simulink library "batt_packBTMSExampleLib"  (R2023a)
settings: Solver=VariableStepAuto  StartTime=0.0  StopTime=10.0  RelTol=1e-3
libraries: batt_packBTMSExampleLib_lib x12
(part 1 of 2)
settings Model: Creator=jjha  LastModifiedBy=jjha
settings OptimizationCC: ReuseModelBlockBuffer=off

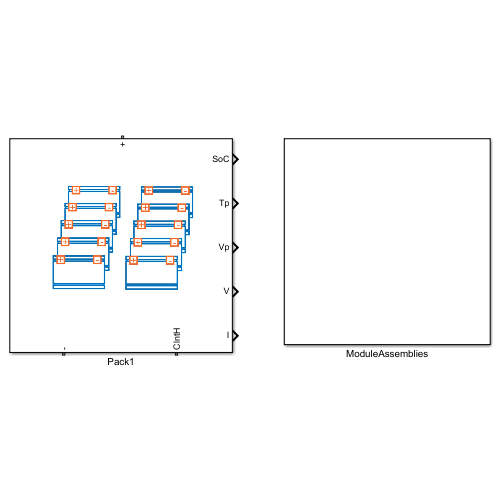
[thumbnail: Simulink's stored preview of the top-level diagram]
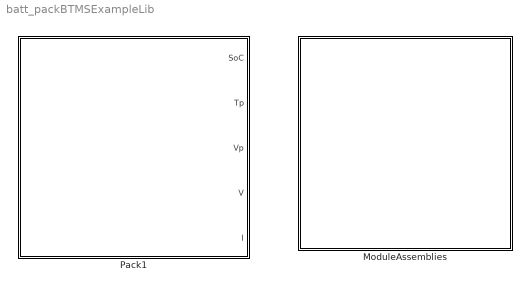
== system batt_packBTMSExampleLib ==
  ModuleAssemblies : Subsystem
  Pack1 : Subsystem
      settings: CopyFcn=set_param(gcb, 'LinkStatus', 'breakWithoutHierarchy')  PortSchema="{\"entries\":[{\"content\":{\"sides\":[{\"content\":{\"connectorIds\":[\"LConn1\"]},\"type\":\"ConnectorPlacement.EquallySpacedRectSide\",\"uuid\":\"7b46babc-8b83-451b-8519-1d7c62ae3771\"},{\"content\":{\"connectorIds\":[\"RConn1\",\"RConn2\"],\"side\":\"RIGHT\"},\"type\":\"ConnectorPlacement.EquallySpacedRectSide\",\"uuid\":\"75c1bf7b-5e52-4279-86bf-85530d236c02\"},{\"content\":{\"connectorIds\":[],\"side\":\"TOP\"},\"type\":\"ConnectorPlacement.EquallySpacedRectSide\",\"uuid\":\"90212396-c9c9-431a-bb2e-a5c41a4990d7\"},{\"content\":{\"connectorIds\":[\"Out1\",\"Out2\",\"Out3\",\"Out4\",\"Out5\"],\"side\":\"BOTTOM\"},\"type\":\"ConnectorPlacement.EquallySpacedRectSide\",\"uuid\":\"256631cd-ebba-4ea5-bbad-0309b84a78ed\"}]},\"type\":\"ConnectorPlacement.EquallySpacedConnector\",\"uuid\":\"fb66d0bc-bd1f-4bb9-a18e-b6b74cdcb9a0\"}],\"packageUris\":[\"http://schema.mathworks.com/mf0/Connector/R2020b\"],\"version\":\"1.0\"}"
      mask Display: image('$imagefile')

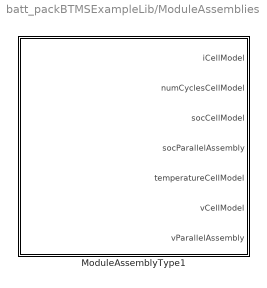
== system batt_packBTMSExampleLib/ModuleAssemblies ==
  ModuleAssemblyType1 : Subsystem
      settings: CopyFcn=set_param(gcb, 'LinkStatus', 'breakWithoutHierarchy')  PortSchema="{\"entries\":[{\"content\":{\"sides\":[{\"content\":{\"connectorIds\":[\"LConn1\"]},\"type\":\"ConnectorPlacement.EquallySpacedRectSide\",\"uuid\":\"7b46babc-8b83-451b-8519-1d7c62ae3771\"},{\"content\":{\"connectorIds\":[\"RConn1\",\"RConn2\"],\"side\":\"RIGHT\"},\"type\":\"ConnectorPlacement.EquallySpacedRectSide\",\"uuid\":\"75c1bf7b-5e52-4279-86bf-85530d236c02\"},{\"content\":{\"connectorIds\":[],\"side\":\"TOP\"},\"type\":\"ConnectorPlacement.EquallySpacedRectSide\",\"uuid\":\"90212396-c9c9-431a-bb2e-a5c41a4990d7\"},{\"content\":{\"connectorIds\":[\"Out1\",\"Out2\",\"Out3\",\"Out4\",\"Out5\",\"Out6\",\"Out7\"],\"side\":\"BOTTOM\"},\"type\":\"ConnectorPlacement.EquallySpacedRectSide\",\"uuid\":\"06be32c4-8297-416c-9a62-5fc7a23f864d\"}]},\"type\":\"ConnectorPlacement.EquallySpacedConnector\",\"uuid\":\"fb66d0bc-bd1f-4bb9-a18e-b6b74cdcb9a0\"}],\"packageUris\":[\"http://schema.mathworks.com/mf0/Connector/R2020b\"],\"version\":\"1.0\"}"
      mask Display: image('$imagefile')

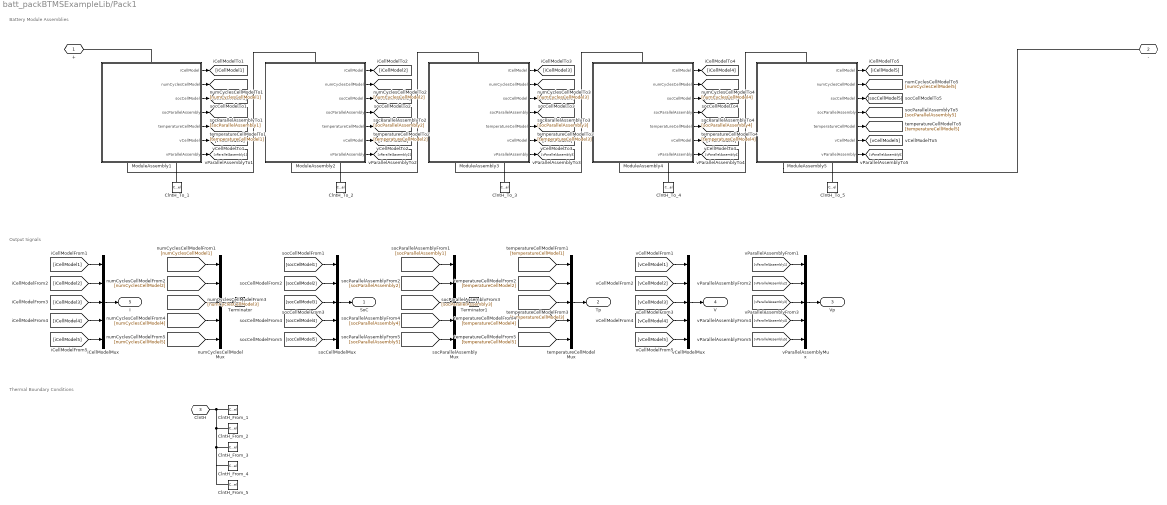
== system batt_packBTMSExampleLib/Pack1 ==
  note: Battery Module Assemblies
  note: Output Signals
  note: Thermal Boundary Conditions
  ClntH_From_1 : ConnectionLabel  Label=clntH_1
  ClntH_From_2 : ConnectionLabel  Label=clntH_2
  ClntH_From_3 : ConnectionLabel  Label=clntH_3
  ClntH_From_4 : ConnectionLabel  Label=clntH_4
  ClntH_From_5 : ConnectionLabel  Label=clntH_5
  ClntH_To_1 : ConnectionLabel  Label=clntH_1
  ClntH_To_2 : ConnectionLabel  Label=clntH_2
  ClntH_To_3 : ConnectionLabel  Label=clntH_3
  ClntH_To_4 : ConnectionLabel  Label=clntH_4
  ClntH_To_5 : ConnectionLabel  Label=clntH_5
  ModuleAssembly1 : Subsystem
      settings: CopyFcn=set_param(gcb, 'LinkStatus', 'breakWithoutHierarchy')  PortSchema="{\"entries\":[{\"content\":{\"sides\":[{\"content\":{\"connectorIds\":[\"LConn1\"]},\"type\":\"ConnectorPlacement.EquallySpacedRectSide\",\"uuid\":\"7b46babc-8b83-451b-8519-1d7c62ae3771\"},{\"content\":{\"connectorIds\":[\"RConn1\",\"RConn2\"],\"side\":\"RIGHT\"},\"type\":\"ConnectorPlacement.EquallySpacedRectSide\",\"uuid\":\"75c1bf7b-5e52-4279-86bf-85530d236c02\"},{\"content\":{\"connectorIds\":[],\"side\":\"TOP\"},\"type\":\"ConnectorPlacement.EquallySpacedRectSide\",\"uuid\":\"90212396-c9c9-431a-bb2e-a5c41a4990d7\"},{\"content\":{\"connectorIds\":[\"Out1\",\"Out2\",\"Out3\",\"Out4\",\"Out5\",\"Out6\",\"Out7\"],\"side\":\"BOTTOM\"},\"type\":\"ConnectorPlacement.EquallySpacedRectSide\",\"uuid\":\"06be32c4-8297-416c-9a62-5fc7a23f864d\"}]},\"type\":\"ConnectorPlacement.EquallySpacedConnector\",\"uuid\":\"fb66d0bc-bd1f-4bb9-a18e-b6b74cdcb9a0\"}],\"packageUris\":[\"http://schema.mathworks.com/mf0/Connector/R2020b\"],\"version\":\"1.0\"}"
      mask Display: image('$imagefile')
  ModuleAssembly2 : Subsystem
      settings: CopyFcn=set_param(gcb, 'LinkStatus', 'breakWithoutHierarchy')  PortSchema="{\"entries\":[{\"content\":{\"sides\":[{\"content\":{\"connectorIds\":[\"LConn1\"]},\"type\":\"ConnectorPlacement.EquallySpacedRectSide\",\"uuid\":\"7b46babc-8b83-451b-8519-1d7c62ae3771\"},{\"content\":{\"connectorIds\":[\"RConn1\",\"RConn2\"],\"side\":\"RIGHT\"},\"type\":\"ConnectorPlacement.EquallySpacedRectSide\",\"uuid\":\"75c1bf7b-5e52-4279-86bf-85530d236c02\"},{\"content\":{\"connectorIds\":[],\"side\":\"TOP\"},\"type\":\"ConnectorPlacement.EquallySpacedRectSide\",\"uuid\":\"90212396-c9c9-431a-bb2e-a5c41a4990d7\"},{\"content\":{\"connectorIds\":[\"Out1\",\"Out2\",\"Out3\",\"Out4\",\"Out5\",\"Out6\",\"Out7\"],\"side\":\"BOTTOM\"},\"type\":\"ConnectorPlacement.EquallySpacedRectSide\",\"uuid\":\"06be32c4-8297-416c-9a62-5fc7a23f864d\"}]},\"type\":\"ConnectorPlacement.EquallySpacedConnector\",\"uuid\":\"fb66d0bc-bd1f-4bb9-a18e-b6b74cdcb9a0\"}],\"packageUris\":[\"http://schema.mathworks.com/mf0/Connector/R2020b\"],\"version\":\"1.0\"}"
      mask Display: image('$imagefile')
  ModuleAssembly3 : Subsystem
      settings: CopyFcn=set_param(gcb, 'LinkStatus', 'breakWithoutHierarchy')  PortSchema="{\"entries\":[{\"content\":{\"sides\":[{\"content\":{\"connectorIds\":[\"LConn1\"]},\"type\":\"ConnectorPlacement.EquallySpacedRectSide\",\"uuid\":\"7b46babc-8b83-451b-8519-1d7c62ae3771\"},{\"content\":{\"connectorIds\":[\"RConn1\",\"RConn2\"],\"side\":\"RIGHT\"},\"type\":\"ConnectorPlacement.EquallySpacedRectSide\",\"uuid\":\"75c1bf7b-5e52-4279-86bf-85530d236c02\"},{\"content\":{\"connectorIds\":[],\"side\":\"TOP\"},\"type\":\"ConnectorPlacement.EquallySpacedRectSide\",\"uuid\":\"90212396-c9c9-431a-bb2e-a5c41a4990d7\"},{\"content\":{\"connectorIds\":[\"Out1\",\"Out2\",\"Out3\",\"Out4\",\"Out5\",\"Out6\",\"Out7\"],\"side\":\"BOTTOM\"},\"type\":\"ConnectorPlacement.EquallySpacedRectSide\",\"uuid\":\"06be32c4-8297-416c-9a62-5fc7a23f864d\"}]},\"type\":\"ConnectorPlacement.EquallySpacedConnector\",\"uuid\":\"fb66d0bc-bd1f-4bb9-a18e-b6b74cdcb9a0\"}],\"packageUris\":[\"http://schema.mathworks.com/mf0/Connector/R2020b\"],\"version\":\"1.0\"}"
      mask Display: image('$imagefile')
  ModuleAssembly4 : Subsystem
      settings: CopyFcn=set_param(gcb, 'LinkStatus', 'breakWithoutHierarchy')  PortSchema="{\"entries\":[{\"content\":{\"sides\":[{\"content\":{\"connectorIds\":[\"LConn1\"]},\"type\":\"ConnectorPlacement.EquallySpacedRectSide\",\"uuid\":\"7b46babc-8b83-451b-8519-1d7c62ae3771\"},{\"content\":{\"connectorIds\":[\"RConn1\",\"RConn2\"],\"side\":\"RIGHT\"},\"type\":\"ConnectorPlacement.EquallySpacedRectSide\",\"uuid\":\"75c1bf7b-5e52-4279-86bf-85530d236c02\"},{\"content\":{\"connectorIds\":[],\"side\":\"TOP\"},\"type\":\"ConnectorPlacement.EquallySpacedRectSide\",\"uuid\":\"90212396-c9c9-431a-bb2e-a5c41a4990d7\"},{\"content\":{\"connectorIds\":[\"Out1\",\"Out2\",\"Out3\",\"Out4\",\"Out5\",\"Out6\",\"Out7\"],\"side\":\"BOTTOM\"},\"type\":\"ConnectorPlacement.EquallySpacedRectSide\",\"uuid\":\"06be32c4-8297-416c-9a62-5fc7a23f864d\"}]},\"type\":\"ConnectorPlacement.EquallySpacedConnector\",\"uuid\":\"fb66d0bc-bd1f-4bb9-a18e-b6b74cdcb9a0\"}],\"packageUris\":[\"http://schema.mathworks.com/mf0/Connector/R2020b\"],\"version\":\"1.0\"}"
      mask Display: image('$imagefile')
  ModuleAssembly5 : Subsystem
      settings: CopyFcn=set_param(gcb, 'LinkStatus', 'breakWithoutHierarchy')  PortSchema="{\"entries\":[{\"content\":{\"sides\":[{\"content\":{\"connectorIds\":[\"LConn1\"]},\"type\":\"ConnectorPlacement.EquallySpacedRectSide\",\"uuid\":\"7b46babc-8b83-451b-8519-1d7c62ae3771\"},{\"content\":{\"connectorIds\":[\"RConn1\",\"RConn2\"],\"side\":\"RIGHT\"},\"type\":\"ConnectorPlacement.EquallySpacedRectSide\",\"uuid\":\"75c1bf7b-5e52-4279-86bf-85530d236c02\"},{\"content\":{\"connectorIds\":[],\"side\":\"TOP\"},\"type\":\"ConnectorPlacement.EquallySpacedRectSide\",\"uuid\":\"90212396-c9c9-431a-bb2e-a5c41a4990d7\"},{\"content\":{\"connectorIds\":[\"Out1\",\"Out2\",\"Out3\",\"Out4\",\"Out5\",\"Out6\",\"Out7\"],\"side\":\"BOTTOM\"},\"type\":\"ConnectorPlacement.EquallySpacedRectSide\",\"uuid\":\"06be32c4-8297-416c-9a62-5fc7a23f864d\"}]},\"type\":\"ConnectorPlacement.EquallySpacedConnector\",\"uuid\":\"fb66d0bc-bd1f-4bb9-a18e-b6b74cdcb9a0\"}],\"packageUris\":[\"http://schema.mathworks.com/mf0/Connector/R2020b\"],\"version\":\"1.0\"}"
      mask Display: image('$imagefile')
  Terminator : Terminator
  Terminator1 : Terminator
  iCellModelMux : Mux  Inputs=5
  numCyclesCellModelMux : Mux  Inputs=5
  socCellModelMux : Mux  Inputs=5
  socParallelAssemblyMux : Mux  Inputs=5
  temperatureCellModelMux : Mux  Inputs=5
  vCellModelMux : Mux  Inputs=5
  vParallelAssemblyMux : Mux  Inputs=5
  + : PMIOPort  Side=Left
  - : PMIOPort  Port=2  Side=Right
  ClntH : PMIOPort  Port=3  Side=Right  ConnectionType=Connection: foundation.thermal.thermal
  SoC : Outport
  Tp : Outport  Port=2
  Vp : Outport  Port=3
  V : Outport  Port=4
  I : Outport  Port=5
  wires:
  ModuleAssembly1/1(iCellModel) -> [iCellModel1]
  iCellModelMux/1 -> I/1
  [iCellModel1] -> iCellModelMux/1
  ModuleAssembly1/2(numCyclesCellModel) -> [numCyclesCellModel1]
  numCyclesCellModelMux/1 -> Terminator/1
  [numCyclesCellModel1] -> numCyclesCellModelMux/1
  ModuleAssembly1/3(socCellModel) -> [socCellModel1]
  socCellModelMux/1 -> SoC/1
  [socCellModel1] -> socCellModelMux/1
  ModuleAssembly1/4(socParallelAssembly) -> [socParallelAssembly1]
  socParallelAssemblyMux/1 -> Terminator1/1
  [socParallelAssembly1] -> socParallelAssemblyMux/1
  ModuleAssembly1/5(temperatureCellModel) -> [temperatureCellModel1]
  temperatureCellModelMux/1 -> Tp/1
  [temperatureCellModel1] -> temperatureCellModelMux/1
  ModuleAssembly1/6(vCellModel) -> [vCellModel1]
  vCellModelMux/1 -> V/1
  [vCellModel1] -> vCellModelMux/1
  ModuleAssembly1/7(vParallelAssembly) -> [vParallelAssembly1]
  vParallelAssemblyMux/1 -> Vp/1
  [vParallelAssembly1] -> vParallelAssemblyMux/1
  ModuleAssembly2/1(iCellModel) -> [iCellModel2]
  [iCellModel2] -> iCellModelMux/2
  ModuleAssembly2/2(numCyclesCellModel) -> [numCyclesCellModel2]
  [numCyclesCellModel2] -> numCyclesCellModelMux/2
  ModuleAssembly2/3(socCellModel) -> [socCellModel2]
  [socCellModel2] -> socCellModelMux/2
  ModuleAssembly2/4(socParallelAssembly) -> [socParallelAssembly2]
  [socParallelAssembly2] -> socParallelAssemblyMux/2
  ModuleAssembly2/5(temperatureCellModel) -> [temperatureCellModel2]
  [temperatureCellModel2] -> temperatureCellModelMux/2
  ModuleAssembly2/6(vCellModel) -> [vCellModel2]
  [vCellModel2] -> vCellModelMux/2
  ModuleAssembly2/7(vParallelAssembly) -> [vParallelAssembly2]
  [vParallelAssembly2] -> vParallelAssemblyMux/2
  ModuleAssembly3/1(iCellModel) -> [iCellModel3]
  [iCellModel3] -> iCellModelMux/3
  ModuleAssembly3/2(numCyclesCellModel) -> [numCyclesCellModel3]
  [numCyclesCellModel3] -> numCyclesCellModelMux/3
  ModuleAssembly3/3(socCellModel) -> [socCellModel3]
  [socCellModel3] -> socCellModelMux/3
  ModuleAssembly3/4(socParallelAssembly) -> [socParallelAssembly3]
  [socParallelAssembly3] -> socParallelAssemblyMux/3
  ModuleAssembly3/5(temperatureCellModel) -> [temperatureCellModel3]
  [temperatureCellModel3] -> temperatureCellModelMux/3
  ModuleAssembly3/6(vCellModel) -> [vCellModel3]
  [vCellModel3] -> vCellModelMux/3
  ModuleAssembly3/7(vParallelAssembly) -> [vParallelAssembly3]
  [vParallelAssembly3] -> vParallelAssemblyMux/3
  ModuleAssembly4/1(iCellModel) -> [iCellModel4]
  [iCellModel4] -> iCellModelMux/4
  ModuleAssembly4/2(numCyclesCellModel) -> [numCyclesCellModel4]
  [numCyclesCellModel4] -> numCyclesCellModelMux/4
  ModuleAssembly4/3(socCellModel) -> [socCellModel4]
  [socCellModel4] -> socCellModelMux/4
  ModuleAssembly4/4(socParallelAssembly) -> [socParallelAssembly4]
  [socParallelAssembly4] -> socParallelAssemblyMux/4
  ModuleAssembly4/5(temperatureCellModel) -> [temperatureCellModel4]
  [temperatureCellModel4] -> temperatureCellModelMux/4
  ModuleAssembly4/6(vCellModel) -> [vCellModel4]
  [vCellModel4] -> vCellModelMux/4
  ModuleAssembly4/7(vParallelAssembly) -> [vParallelAssembly4]
  [vParallelAssembly4] -> vParallelAssemblyMux/4
  ModuleAssembly5/1(iCellModel) -> [iCellModel5]
  [iCellModel5] -> iCellModelMux/5
  ModuleAssembly5/2(numCyclesCellModel) -> [numCyclesCellModel5]
  [numCyclesCellModel5] -> numCyclesCellModelMux/5
  ModuleAssembly5/3(socCellModel) -> [socCellModel5]
  [socCellModel5] -> socCellModelMux/5
  ModuleAssembly5/4(socParallelAssembly) -> [socParallelAssembly5]
  [socParallelAssembly5] -> socParallelAssemblyMux/5
  ModuleAssembly5/5(temperatureCellModel) -> [temperatureCellModel5]
  [temperatureCellModel5] -> temperatureCellModelMux/5
  ModuleAssembly5/6(vCellModel) -> [vCellModel5]
  [vCellModel5] -> vCellModelMux/5
  ModuleAssembly5/7(vParallelAssembly) -> [vParallelAssembly5]
  [vParallelAssembly5] -> vParallelAssemblyMux/5
  connections:
  ModuleAssembly2/LConn1 -- ModuleAssembly1/RConn1
  ModuleAssembly3/LConn1 -- ModuleAssembly2/RConn1
  ModuleAssembly4/LConn1 -- ModuleAssembly3/RConn1
  ModuleAssembly5/LConn1 -- ModuleAssembly4/RConn1
  ModuleAssembly1/LConn1 -- +/RConn1
  ModuleAssembly5/RConn1 -- -/RConn1
  ClntH_To_1/LConn1 -- ModuleAssembly1/RConn2
  ClntH_From_1/LConn1 -- ClntH_From_5/LConn1 -- ClntH_From_4/LConn1 -- ClntH_From_3/LConn1 -- ClntH_From_2/LConn1 -- ClntH/RConn1
  ClntH_To_2/LConn1 -- ModuleAssembly2/RConn2
  ClntH_To_3/LConn1 -- ModuleAssembly3/RConn2
  ClntH_To_4/LConn1 -- ModuleAssembly4/RConn2
  ClntH_To_5/LConn1 -- ModuleAssembly5/RConn2

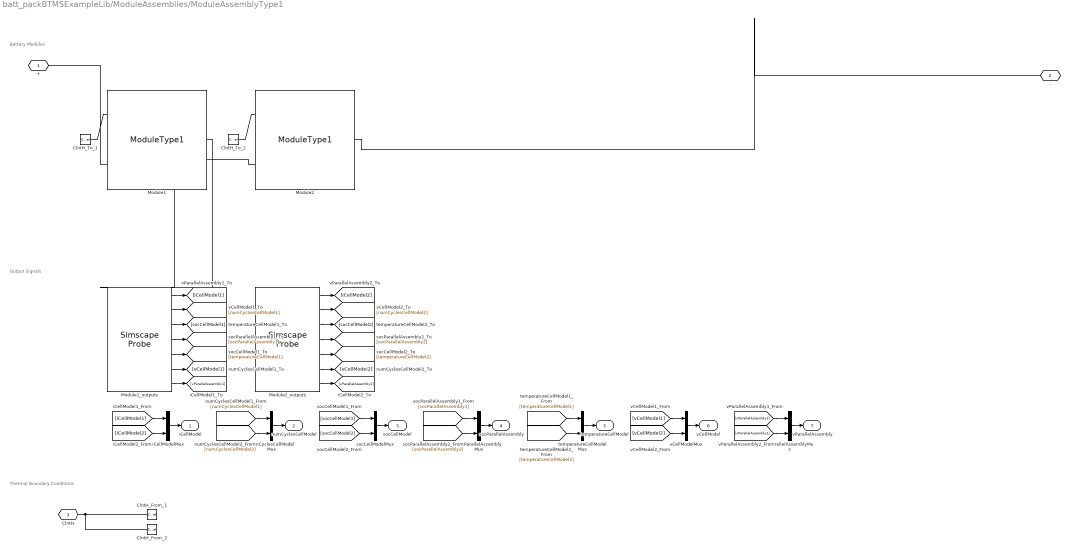
== system batt_packBTMSExampleLib/ModuleAssemblies/ModuleAssemblyType1 ==
  note: Battery Modules
  note: Output Signals
  note: Thermal Boundary Conditions
  ClntH_From_1 : ConnectionLabel  Label=clntH_1
  ClntH_From_2 : ConnectionLabel  Label=clntH_2
  ClntH_To_1 : ConnectionLabel  Label=clntH_1
  ClntH_To_2 : ConnectionLabel  Label=clntH_2
  Module1 : batt_packBTMSExampleLib_lib/Modules/ModuleType1  SOC_vec=ModuleType1.SOC_vec  T_vec=ModuleType1.T_vec K  V0_mat=ModuleType1.V0_mat V  V_range=ModuleType1.V_range V  R0_mat=ModuleType1.R0_mat Ohm  AH=ModuleType1.AH A*hr  extrapolation_option=simscape.enum.extrapolation.nearest  thermal_mass=ModuleType1.thermal_mass J/K  CoolantThermalPathResistance=ModuleType1.CoolantThermalPathResistance K/W  P=3  S=11  iCellModel_specify=off  iCellModel_priority=None  iCellModel=0 A  iCellModel_nominal_specify=off  iCellModel_nominal_unit=A  iCellModel_nominal_value=1  vCellModel_specify=off  vCellModel_priority=None  vCellModel=0 V  vCellModel_nominal_specify=off  vCellModel_nominal_unit=V  vCellModel_nominal_value=1  socCellModel_specify=off  socCellModel_priority=High  socCellModel=1  socCellModel_nominal_specify=off  socCellModel_nominal_unit=1  socCellModel_nominal_value=1  numCyclesCellModel_specify=off  numCyclesCellModel_priority=High  numCyclesCellModel=0  numCyclesCellModel_nominal_specify=off  numCyclesCellModel_nominal_unit=1  numCyclesCellModel_nominal_value=1  temperatureCellModel_specify=off  temperatureCellModel_priority=High  temperatureCellModel=298.15 K  temperatureCellModel_nominal_specify=off  temperatureCellModel_nominal_unit=K  temperatureCellModel_nominal_value=1  vParallelAssembly_specify=off  vParallelAssembly_priority=None  vParallelAssembly=repmat(0, 11, 1) V  vParallelAssembly_nominal_specify=off  vParallelAssembly_nominal_unit=V  vParallelAssembly_nominal_value=1  socParallelAssembly_specify=off  socParallelAssembly_priority=None  socParallelAssembly=repmat(1, 11, 1)  socParallelAssembly_nominal_specify=off  socParallelAssembly_nominal_unit=1  socParallelAssembly_nominal_value=1
      settings: InternalSimscapePortConfiguration="{\"Bottom\":[{\"id\":\"n\",\"label\":\"-\",\"type\":\"foundation.electrical.electrical\"}],\"Left\":[{\"id\":\"ClntH\",\"label\":\"CH\",\"type\":\"foundation.thermal.thermal\"}],\"Right\":[],\"Top\":[{\"id\":\"p\",\"label\":\"+\",\"type\":\"foundation.electrical.electrical\"}]}"
  Module1_outputs : SimscapeProbe  BoundBlock=3  Variables={iCellModel, numCyclesCellModel, socCellModel, socParallelAssembly, temperatureCellModel, vCellModel, vParallelAssembly}
  Module2 : batt_packBTMSExampleLib_lib/Modules/ModuleType1  SOC_vec=ModuleType1.SOC_vec  T_vec=ModuleType1.T_vec K  V0_mat=ModuleType1.V0_mat V  V_range=ModuleType1.V_range V  R0_mat=ModuleType1.R0_mat Ohm  AH=ModuleType1.AH A*hr  extrapolation_option=simscape.enum.extrapolation.nearest  thermal_mass=ModuleType1.thermal_mass J/K  CoolantThermalPathResistance=ModuleType1.CoolantThermalPathResistance K/W  P=3  S=11  iCellModel_specify=off  iCellModel_priority=None  iCellModel=0 A  iCellModel_nominal_specify=off  iCellModel_nominal_unit=A  iCellModel_nominal_value=1  vCellModel_specify=off  vCellModel_priority=None  vCellModel=0 V  vCellModel_nominal_specify=off  vCellModel_nominal_unit=V  vCellModel_nominal_value=1  socCellModel_specify=off  socCellModel_priority=High  socCellModel=1  socCellModel_nominal_specify=off  socCellModel_nominal_unit=1  socCellModel_nominal_value=1  numCyclesCellModel_specify=off  numCyclesCellModel_priority=High  numCyclesCellModel=0  numCyclesCellModel_nominal_specify=off  numCyclesCellModel_nominal_unit=1  numCyclesCellModel_nominal_value=1  temperatureCellModel_specify=off  temperatureCellModel_priority=High  temperatureCellModel=298.15 K  temperatureCellModel_nominal_specify=off  temperatureCellModel_nominal_unit=K  temperatureCellModel_nominal_value=1  vParallelAssembly_specify=off  vParallelAssembly_priority=None  vParallelAssembly=repmat(0, 11, 1) V  vParallelAssembly_nominal_specify=off  vParallelAssembly_nominal_unit=V  vParallelAssembly_nominal_value=1  socParallelAssembly_specify=off  socParallelAssembly_priority=None  socParallelAssembly=repmat(1, 11, 1)  socParallelAssembly_nominal_specify=off  socParallelAssembly_nominal_unit=1  socParallelAssembly_nominal_value=1
      settings: InternalSimscapePortConfiguration="{\"Bottom\":[{\"id\":\"n\",\"label\":\"-\",\"type\":\"foundation.electrical.electrical\"}],\"Left\":[{\"id\":\"ClntH\",\"label\":\"CH\",\"type\":\"foundation.thermal.thermal\"}],\"Right\":[],\"Top\":[{\"id\":\"p\",\"label\":\"+\",\"type\":\"foundation.electrical.electrical\"}]}"
  Module2_outputs : SimscapeProbe  BoundBlock=4  Variables={iCellModel, numCyclesCellModel, socCellModel, socParallelAssembly, temperatureCellModel, vCellModel, vParallelAssembly}
  iCellModelMux : Mux  Inputs=2
  numCyclesCellModelMux : Mux  Inputs=2
  socCellModelMux : Mux  Inputs=2
  socParallelAssemblyMux : Mux  Inputs=2
  temperatureCellModelMux : Mux  Inputs=2
  vCellModelMux : Mux  Inputs=2
  vParallelAssemblyMux : Mux  Inputs=2
  + : PMIOPort  Side=Left
  - : PMIOPort  Port=2  Side=Right
  ClntH : PMIOPort  Port=3  Side=Right
  iCellModel : Outport
  numCyclesCellModel : Outport  Port=2
  socCellModel : Outport  Port=3
  socParallelAssembly : Outport  Port=4
  temperatureCellModel : Outport  Port=5
  vCellModel : Outport  Port=6
  vParallelAssembly : Outport  Port=7
  wires:
  Module1_outputs/7 -> [vParallelAssembly1]
  iCellModelMux/1 -> iCellModel/1
  [iCellModel1] -> iCellModelMux/1
  Module1_outputs/6 -> [vCellModel1]
  numCyclesCellModelMux/1 -> numCyclesCellModel/1
  [numCyclesCellModel1] -> numCyclesCellModelMux/1
  Module1_outputs/5 -> [temperatureCellModel1]
  socCellModelMux/1 -> socCellModel/1
  [socCellModel1] -> socCellModelMux/1
  Module1_outputs/4 -> [socParallelAssembly1]
  socParallelAssemblyMux/1 -> socParallelAssembly/1
  [socParallelAssembly1] -> socParallelAssemblyMux/1
  Module1_outputs/3 -> [socCellModel1]
  temperatureCellModelMux/1 -> temperatureCellModel/1
  [temperatureCellModel1] -> temperatureCellModelMux/1
  Module1_outputs/2 -> [numCyclesCellModel1]
  vCellModelMux/1 -> vCellModel/1
  [vCellModel1] -> vCellModelMux/1
  Module1_outputs/1 -> [iCellModel1]
  vParallelAssemblyMux/1 -> vParallelAssembly/1
  [vParallelAssembly1] -> vParallelAssemblyMux/1
  Module2_outputs/7 -> [vParallelAssembly2]
  [iCellModel2] -> iCellModelMux/2
  Module2_outputs/6 -> [vCellModel2]
  [numCyclesCellModel2] -> numCyclesCellModelMux/2
  Module2_outputs/5 -> [temperatureCellModel2]
  [socCellModel2] -> socCellModelMux/2
  Module2_outputs/4 -> [socParallelAssembly2]
  [socParallelAssembly2] -> socParallelAssemblyMux/2
  Module2_outputs/3 -> [socCellModel2]
  [temperatureCellModel2] -> temperatureCellModelMux/2
  Module2_outputs/2 -> [numCyclesCellModel2]
  [vCellModel2] -> vCellModelMux/2
  Module2_outputs/1 -> [iCellModel2]
  [vParallelAssembly2] -> vParallelAssemblyMux/2
  connections:
  Module2/LConn2 -- Module1/RConn1
  Module1/LConn2 -- +/RConn1
  Module2/RConn1 -- -/RConn1
  ClntH_To_1/LConn1 -- Module1/LConn1
  ClntH/RConn1 -- ClntH_From_1/LConn1 -- ClntH_From_2/LConn1
  ClntH_To_2/LConn1 -- Module2/LConn1

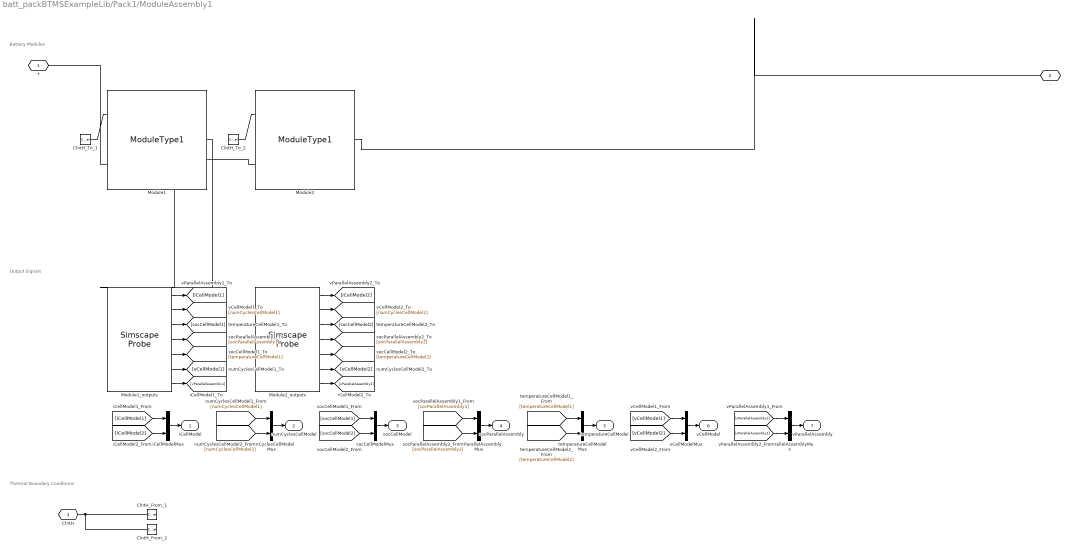
== system batt_packBTMSExampleLib/Pack1/ModuleAssembly1 ==
  note: Thermal Boundary Conditions
  note: Output Signals
  note: Battery Modules
  ClntH_From_1 : ConnectionLabel  Label=clntH_1
  ClntH_From_2 : ConnectionLabel  Label=clntH_2
  ClntH_To_1 : ConnectionLabel  Label=clntH_1
  ClntH_To_2 : ConnectionLabel  Label=clntH_2
  Module1 : batt_packBTMSExampleLib_lib/Modules/ModuleType1  SOC_vec=ModuleType1.SOC_vec  T_vec=ModuleType1.T_vec K  V0_mat=ModuleType1.V0_mat V  V_range=ModuleType1.V_range V  R0_mat=ModuleType1.R0_mat Ohm  AH=ModuleType1.AH A*hr  extrapolation_option=simscape.enum.extrapolation.nearest  thermal_mass=ModuleType1.thermal_mass J/K  CoolantThermalPathResistance=ModuleType1.CoolantThermalPathResistance K/W  P=3  S=11  iCellModel_specify=on  iCellModel_priority=None  iCellModel=ModuleAssembly1.Module1.iCellModel A  iCellModel_nominal_specify=off  iCellModel_nominal_unit=A  iCellModel_nominal_value=1  vCellModel_specify=on  vCellModel_priority=None  vCellModel=ModuleAssembly1.Module1.vCellModel V  vCellModel_nominal_specify=off  vCellModel_nominal_unit=V  vCellModel_nominal_value=1  socCellModel_specify=on  socCellModel_priority=High  socCellModel=ModuleAssembly1.Module1.socCellModel  socCellModel_nominal_specify=off  socCellModel_nominal_unit=1  socCellModel_nominal_value=1  numCyclesCellModel_specify=on  numCyclesCellModel_priority=High  numCyclesCellModel=ModuleAssembly1.Module1.numCyclesCellModel  numCyclesCellModel_nominal_specify=off  numCyclesCellModel_nominal_unit=1  numCyclesCellModel_nominal_value=1  temperatureCellModel_specify=on  temperatureCellModel_priority=High  temperatureCellModel=ModuleAssembly1.Module1.temperatureCellModel K  temperatureCellModel_nominal_specify=off  temperatureCellModel_nominal_unit=K  temperatureCellModel_nominal_value=1  vParallelAssembly_specify=on  vParallelAssembly_priority=None  vParallelAssembly=ModuleAssembly1.Module1.vParallelAssembly V  vParallelAssembly_nominal_specify=off  vParallelAssembly_nominal_unit=V  vParallelAssembly_nominal_value=1  socParallelAssembly_specify=on  socParallelAssembly_priority=None  socParallelAssembly=ModuleAssembly1.Module1.socParallelAssembly  socParallelAssembly_nominal_specify=off  socParallelAssembly_nominal_unit=1  socParallelAssembly_nominal_value=1
      settings: InternalSimscapePortConfiguration="{\"Bottom\":[{\"id\":\"n\",\"label\":\"-\",\"type\":\"foundation.electrical.electrical\"}],\"Left\":[{\"id\":\"ClntH\",\"label\":\"CH\",\"type\":\"foundation.thermal.thermal\"}],\"Right\":[],\"Top\":[{\"id\":\"p\",\"label\":\"+\",\"type\":\"foundation.electrical.electrical\"}]}"
  Module1_outputs : SimscapeProbe  BoundBlock=65  Variables={iCellModel, numCyclesCellModel, socCellModel, socParallelAssembly, temperatureCellModel, vCellModel, vParallelAssembly}
  Module2 : batt_packBTMSExampleLib_lib/Modules/ModuleType1  SOC_vec=ModuleType1.SOC_vec  T_vec=ModuleType1.T_vec K  V0_mat=ModuleType1.V0_mat V  V_range=ModuleType1.V_range V  R0_mat=ModuleType1.R0_mat Ohm  AH=ModuleType1.AH A*hr  extrapolation_option=simscape.enum.extrapolation.nearest  thermal_mass=ModuleType1.thermal_mass J/K  CoolantThermalPathResistance=ModuleType1.CoolantThermalPathResistance K/W  P=3  S=11  iCellModel_specify=on  iCellModel_priority=None  iCellModel=ModuleAssembly1.Module2.iCellModel A  iCellModel_nominal_specify=off  iCellModel_nominal_unit=A  iCellModel_nominal_value=1  vCellModel_specify=on  vCellModel_priority=None  vCellModel=ModuleAssembly1.Module2.vCellModel V  vCellModel_nominal_specify=off  vCellModel_nominal_unit=V  vCellModel_nominal_value=1  socCellModel_specify=on  socCellModel_priority=High  socCellModel=ModuleAssembly1.Module2.socCellModel  socCellModel_nominal_specify=off  socCellModel_nominal_unit=1  socCellModel_nominal_value=1  numCyclesCellModel_specify=on  numCyclesCellModel_priority=High  numCyclesCellModel=ModuleAssembly1.Module2.numCyclesCellModel  numCyclesCellModel_nominal_specify=off  numCyclesCellModel_nominal_unit=1  numCyclesCellModel_nominal_value=1  temperatureCellModel_specify=on  temperatureCellModel_priority=High  temperatureCellModel=ModuleAssembly1.Module2.temperatureCellModel K  temperatureCellModel_nominal_specify=off  temperatureCellModel_nominal_unit=K  temperatureCellModel_nominal_value=1  vParallelAssembly_specify=on  vParallelAssembly_priority=None  vParallelAssembly=ModuleAssembly1.Module2.vParallelAssembly V  vParallelAssembly_nominal_specify=off  vParallelAssembly_nominal_unit=V  vParallelAssembly_nominal_value=1  socParallelAssembly_specify=on  socParallelAssembly_priority=None  socParallelAssembly=ModuleAssembly1.Module2.socParallelAssembly  socParallelAssembly_nominal_specify=off  socParallelAssembly_nominal_unit=1  socParallelAssembly_nominal_value=1
      settings: InternalSimscapePortConfiguration="{\"Bottom\":[{\"id\":\"n\",\"label\":\"-\",\"type\":\"foundation.electrical.electrical\"}],\"Left\":[{\"id\":\"ClntH\",\"label\":\"CH\",\"type\":\"foundation.thermal.thermal\"}],\"Right\":[],\"Top\":[{\"id\":\"p\",\"label\":\"+\",\"type\":\"foundation.electrical.electrical\"}]}"
  Module2_outputs : SimscapeProbe  BoundBlock=67  Variables={iCellModel, numCyclesCellModel, socCellModel, socParallelAssembly, temperatureCellModel, vCellModel, vParallelAssembly}
  iCellModelMux : Mux  Inputs=2
  numCyclesCellModelMux : Mux  Inputs=2
  socCellModelMux : Mux  Inputs=2
  socParallelAssemblyMux : Mux  Inputs=2
  temperatureCellModelMux : Mux  Inputs=2
  vCellModelMux : Mux  Inputs=2
  vParallelAssemblyMux : Mux  Inputs=2
  + : PMIOPort  Side=Left
  - : PMIOPort  Port=2  Side=Right
  ClntH : PMIOPort  Port=3  Side=Right
  iCellModel : Outport
  numCyclesCellModel : Outport  Port=2
  socCellModel : Outport  Port=3
  socParallelAssembly : Outport  Port=4
  temperatureCellModel : Outport  Port=5
  vCellModel : Outport  Port=6
  vParallelAssembly : Outport  Port=7
  wires:
  [vParallelAssembly2] -> vParallelAssemblyMux/2
  Module2_outputs/1 -> [iCellModel2]
  [vCellModel2] -> vCellModelMux/2
  Module2_outputs/2 -> [numCyclesCellModel2]
  [temperatureCellModel2] -> temperatureCellModelMux/2
  Module2_outputs/3 -> [socCellModel2]
  [socParallelAssembly2] -> socParallelAssemblyMux/2
  Module2_outputs/4 -> [socParallelAssembly2]
  [socCellModel2] -> socCellModelMux/2
  Module2_outputs/5 -> [temperatureCellModel2]
  [numCyclesCellModel2] -> numCyclesCellModelMux/2
  Module2_outputs/6 -> [vCellModel2]
  [iCellModel2] -> iCellModelMux/2
  Module2_outputs/7 -> [vParallelAssembly2]
  [vParallelAssembly1] -> vParallelAssemblyMux/1
  vParallelAssemblyMux/1 -> vParallelAssembly/1
  Module1_outputs/1 -> [iCellModel1]
  [vCellModel1] -> vCellModelMux/1
  vCellModelMux/1 -> vCellModel/1
  Module1_outputs/2 -> [numCyclesCellModel1]
  [temperatureCellModel1] -> temperatureCellModelMux/1
  temperatureCellModelMux/1 -> temperatureCellModel/1
  Module1_outputs/3 -> [socCellModel1]
  [socParallelAssembly1] -> socParallelAssemblyMux/1
  socParallelAssemblyMux/1 -> socParallelAssembly/1
  Module1_outputs/4 -> [socParallelAssembly1]
  [socCellModel1] -> socCellModelMux/1
  socCellModelMux/1 -> socCellModel/1
  Module1_outputs/5 -> [temperatureCellModel1]
  [numCyclesCellModel1] -> numCyclesCellModelMux/1
  numCyclesCellModelMux/1 -> numCyclesCellModel/1
  Module1_outputs/6 -> [vCellModel1]
  [iCellModel1] -> iCellModelMux/1
  iCellModelMux/1 -> iCellModel/1
  Module1_outputs/7 -> [vParallelAssembly1]
  connections:
  ClntH_To_2/LConn1 -- Module2/LConn1
  ClntH_From_2/LConn1 -- ClntH_From_1/LConn1 -- ClntH/RConn1
  ClntH_To_1/LConn1 -- Module1/LConn1
  Module2/RConn1 -- -/RConn1
  Module1/LConn2 -- +/RConn1
  Module2/LConn2 -- Module1/RConn1

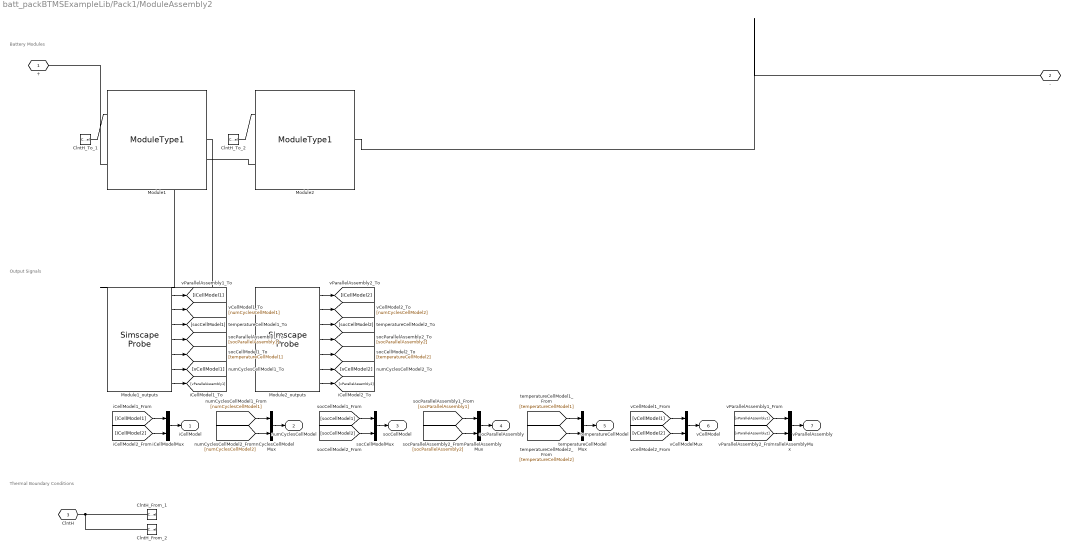
== system batt_packBTMSExampleLib/Pack1/ModuleAssembly2 ==
  note: Thermal Boundary Conditions
  note: Output Signals
  note: Battery Modules
  ClntH_From_1 : ConnectionLabel  Label=clntH_1
  ClntH_From_2 : ConnectionLabel  Label=clntH_2
  ClntH_To_1 : ConnectionLabel  Label=clntH_1
  ClntH_To_2 : ConnectionLabel  Label=clntH_2
  Module1 : batt_packBTMSExampleLib_lib/Modules/ModuleType1  SOC_vec=ModuleType1.SOC_vec  T_vec=ModuleType1.T_vec K  V0_mat=ModuleType1.V0_mat V  V_range=ModuleType1.V_range V  R0_mat=ModuleType1.R0_mat Ohm  AH=ModuleType1.AH A*hr  extrapolation_option=simscape.enum.extrapolation.nearest  thermal_mass=ModuleType1.thermal_mass J/K  CoolantThermalPathResistance=ModuleType1.CoolantThermalPathResistance K/W  P=3  S=11  iCellModel_specify=on  iCellModel_priority=None  iCellModel=ModuleAssembly2.Module1.iCellModel A  iCellModel_nominal_specify=off  iCellModel_nominal_unit=A  iCellModel_nominal_value=1  vCellModel_specify=on  vCellModel_priority=None  vCellModel=ModuleAssembly2.Module1.vCellModel V  vCellModel_nominal_specify=off  vCellModel_nominal_unit=V  vCellModel_nominal_value=1  socCellModel_specify=on  socCellModel_priority=High  socCellModel=ModuleAssembly2.Module1.socCellModel  socCellModel_nominal_specify=off  socCellModel_nominal_unit=1  socCellModel_nominal_value=1  numCyclesCellModel_specify=on  numCyclesCellModel_priority=High  numCyclesCellModel=ModuleAssembly2.Module1.numCyclesCellModel  numCyclesCellModel_nominal_specify=off  numCyclesCellModel_nominal_unit=1  numCyclesCellModel_nominal_value=1  temperatureCellModel_specify=on  temperatureCellModel_priority=High  temperatureCellModel=ModuleAssembly2.Module1.temperatureCellModel K  temperatureCellModel_nominal_specify=off  temperatureCellModel_nominal_unit=K  temperatureCellModel_nominal_value=1  vParallelAssembly_specify=on  vParallelAssembly_priority=None  vParallelAssembly=ModuleAssembly2.Module1.vParallelAssembly V  vParallelAssembly_nominal_specify=off  vParallelAssembly_nominal_unit=V  vParallelAssembly_nominal_value=1  socParallelAssembly_specify=on  socParallelAssembly_priority=None  socParallelAssembly=ModuleAssembly2.Module1.socParallelAssembly  socParallelAssembly_nominal_specify=off  socParallelAssembly_nominal_unit=1  socParallelAssembly_nominal_value=1
      settings: InternalSimscapePortConfiguration="{\"Bottom\":[{\"id\":\"n\",\"label\":\"-\",\"type\":\"foundation.electrical.electrical\"}],\"Left\":[{\"id\":\"ClntH\",\"label\":\"CH\",\"type\":\"foundation.thermal.thermal\"}],\"Right\":[],\"Top\":[{\"id\":\"p\",\"label\":\"+\",\"type\":\"foundation.electrical.electrical\"}]}"
  Module1_outputs : SimscapeProbe  BoundBlock=122  Variables={iCellModel, numCyclesCellModel, socCellModel, socParallelAssembly, temperatureCellModel, vCellModel, vParallelAssembly}
  Module2 : batt_packBTMSExampleLib_lib/Modules/ModuleType1  SOC_vec=ModuleType1.SOC_vec  T_vec=ModuleType1.T_vec K  V0_mat=ModuleType1.V0_mat V  V_range=ModuleType1.V_range V  R0_mat=ModuleType1.R0_mat Ohm  AH=ModuleType1.AH A*hr  extrapolation_option=simscape.enum.extrapolation.nearest  thermal_mass=ModuleType1.thermal_mass J/K  CoolantThermalPathResistance=ModuleType1.CoolantThermalPathResistance K/W  P=3  S=11  iCellModel_specify=on  iCellModel_priority=None  iCellModel=ModuleAssembly2.Module2.iCellModel A  iCellModel_nominal_specify=off  iCellModel_nominal_unit=A  iCellModel_nominal_value=1  vCellModel_specify=on  vCellModel_priority=None  vCellModel=ModuleAssembly2.Module2.vCellModel V  vCellModel_nominal_specify=off  vCellModel_nominal_unit=V  vCellModel_nominal_value=1  socCellModel_specify=on  socCellModel_priority=High  socCellModel=ModuleAssembly2.Module2.socCellModel  socCellModel_nominal_specify=off  socCellModel_nominal_unit=1  socCellModel_nominal_value=1  numCyclesCellModel_specify=on  numCyclesCellModel_priority=High  numCyclesCellModel=ModuleAssembly2.Module2.numCyclesCellModel  numCyclesCellModel_nominal_specify=off  numCyclesCellModel_nominal_unit=1  numCyclesCellModel_nominal_value=1  temperatureCellModel_specify=on  temperatureCellModel_priority=High  temperatureCellModel=ModuleAssembly2.Module2.temperatureCellModel K  temperatureCellModel_nominal_specify=off  temperatureCellModel_nominal_unit=K  temperatureCellModel_nominal_value=1  vParallelAssembly_specify=on  vParallelAssembly_priority=None  vParallelAssembly=ModuleAssembly2.Module2.vParallelAssembly V  vParallelAssembly_nominal_specify=off  vParallelAssembly_nominal_unit=V  vParallelAssembly_nominal_value=1  socParallelAssembly_specify=on  socParallelAssembly_priority=None  socParallelAssembly=ModuleAssembly2.Module2.socParallelAssembly  socParallelAssembly_nominal_specify=off  socParallelAssembly_nominal_unit=1  socParallelAssembly_nominal_value=1
      settings: InternalSimscapePortConfiguration="{\"Bottom\":[{\"id\":\"n\",\"label\":\"-\",\"type\":\"foundation.electrical.electrical\"}],\"Left\":[{\"id\":\"ClntH\",\"label\":\"CH\",\"type\":\"foundation.thermal.thermal\"}],\"Right\":[],\"Top\":[{\"id\":\"p\",\"label\":\"+\",\"type\":\"foundation.electrical.electrical\"}]}"
  Module2_outputs : SimscapeProbe  BoundBlock=124  Variables={iCellModel, numCyclesCellModel, socCellModel, socParallelAssembly, temperatureCellModel, vCellModel, vParallelAssembly}
  iCellModelMux : Mux  Inputs=2
  numCyclesCellModelMux : Mux  Inputs=2
  socCellModelMux : Mux  Inputs=2
  socParallelAssemblyMux : Mux  Inputs=2
  temperatureCellModelMux : Mux  Inputs=2
  vCellModelMux : Mux  Inputs=2
  vParallelAssemblyMux : Mux  Inputs=2
  + : PMIOPort  Side=Left
  - : PMIOPort  Port=2  Side=Right
  ClntH : PMIOPort  Port=3  Side=Right
  iCellModel : Outport
  numCyclesCellModel : Outport  Port=2
  socCellModel : Outport  Port=3
  socParallelAssembly : Outport  Port=4
  temperatureCellModel : Outport  Port=5
  vCellModel : Outport  Port=6
  vParallelAssembly : Outport  Port=7
  wires:
  [vParallelAssembly2] -> vParallelAssemblyMux/2
  Module2_outputs/1 -> [iCellModel2]
  [vCellModel2] -> vCellModelMux/2
  Module2_outputs/2 -> [numCyclesCellModel2]
  [temperatureCellModel2] -> temperatureCellModelMux/2
  Module2_outputs/3 -> [socCellModel2]
  [socParallelAssembly2] -> socParallelAssemblyMux/2
  Module2_outputs/4 -> [socParallelAssembly2]
  [socCellModel2] -> socCellModelMux/2
  Module2_outputs/5 -> [temperatureCellModel2]
  [numCyclesCellModel2] -> numCyclesCellModelMux/2
  Module2_outputs/6 -> [vCellModel2]
  [iCellModel2] -> iCellModelMux/2
  Module2_outputs/7 -> [vParallelAssembly2]
  [vParallelAssembly1] -> vParallelAssemblyMux/1
  vParallelAssemblyMux/1 -> vParallelAssembly/1
  Module1_outputs/1 -> [iCellModel1]
  [vCellModel1] -> vCellModelMux/1
  vCellModelMux/1 -> vCellModel/1
  Module1_outputs/2 -> [numCyclesCellModel1]
  [temperatureCellModel1] -> temperatureCellModelMux/1
  temperatureCellModelMux/1 -> temperatureCellModel/1
  Module1_outputs/3 -> [socCellModel1]
  [socParallelAssembly1] -> socParallelAssemblyMux/1
  socParallelAssemblyMux/1 -> socParallelAssembly/1
  Module1_outputs/4 -> [socParallelAssembly1]
  [socCellModel1] -> socCellModelMux/1
  socCellModelMux/1 -> socCellModel/1
  Module1_outputs/5 -> [temperatureCellModel1]
  [numCyclesCellModel1] -> numCyclesCellModelMux/1
  numCyclesCellModelMux/1 -> numCyclesCellModel/1
  Module1_outputs/6 -> [vCellModel1]
  [iCellModel1] -> iCellModelMux/1
  iCellModelMux/1 -> iCellModel/1
  Module1_outputs/7 -> [vParallelAssembly1]
  connections:
  ClntH_To_2/LConn1 -- Module2/LConn1
  ClntH_From_2/LConn1 -- ClntH_From_1/LConn1 -- ClntH/RConn1
  ClntH_To_1/LConn1 -- Module1/LConn1
  Module2/RConn1 -- -/RConn1
  Module1/LConn2 -- +/RConn1
  Module2/LConn2 -- Module1/RConn1

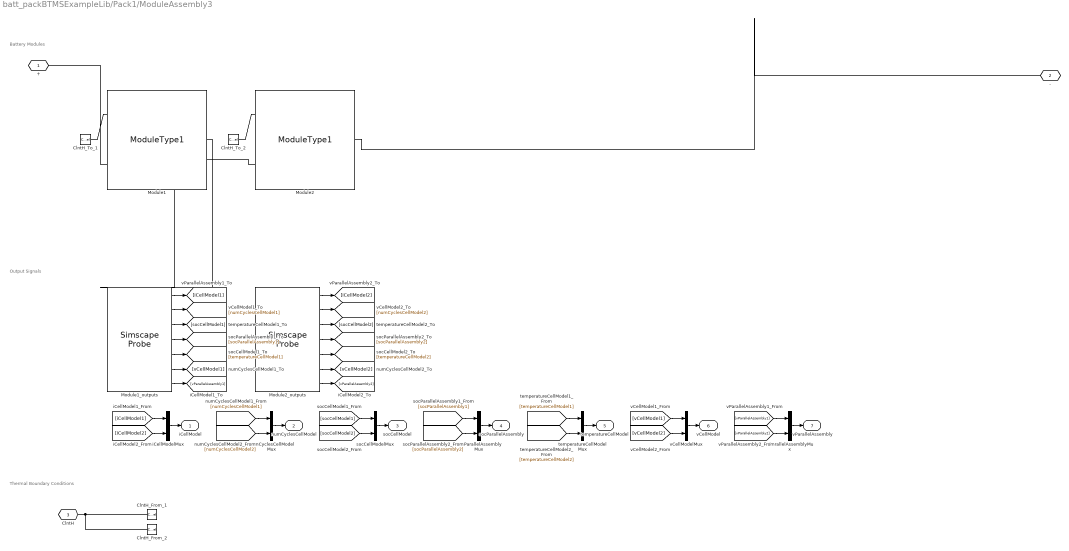
== system batt_packBTMSExampleLib/Pack1/ModuleAssembly3 ==
  note: Thermal Boundary Conditions
  note: Output Signals
  note: Battery Modules
  ClntH_From_1 : ConnectionLabel  Label=clntH_1
  ClntH_From_2 : ConnectionLabel  Label=clntH_2
  ClntH_To_1 : ConnectionLabel  Label=clntH_1
  ClntH_To_2 : ConnectionLabel  Label=clntH_2
  Module1 : batt_packBTMSExampleLib_lib/Modules/ModuleType1  SOC_vec=ModuleType1.SOC_vec  T_vec=ModuleType1.T_vec K  V0_mat=ModuleType1.V0_mat V  V_range=ModuleType1.V_range V  R0_mat=ModuleType1.R0_mat Ohm  AH=ModuleType1.AH A*hr  extrapolation_option=simscape.enum.extrapolation.nearest  thermal_mass=ModuleType1.thermal_mass J/K  CoolantThermalPathResistance=ModuleType1.CoolantThermalPathResistance K/W  P=3  S=11  iCellModel_specify=on  iCellModel_priority=None  iCellModel=ModuleAssembly3.Module1.iCellModel A  iCellModel_nominal_specify=off  iCellModel_nominal_unit=A  iCellModel_nominal_value=1  vCellModel_specify=on  vCellModel_priority=None  vCellModel=ModuleAssembly3.Module1.vCellModel V  vCellModel_nominal_specify=off  vCellModel_nominal_unit=V  vCellModel_nominal_value=1  socCellModel_specify=on  socCellModel_priority=High  socCellModel=ModuleAssembly3.Module1.socCellModel  socCellModel_nominal_specify=off  socCellModel_nominal_unit=1  socCellModel_nominal_value=1  numCyclesCellModel_specify=on  numCyclesCellModel_priority=High  numCyclesCellModel=ModuleAssembly3.Module1.numCyclesCellModel  numCyclesCellModel_nominal_specify=off  numCyclesCellModel_nominal_unit=1  numCyclesCellModel_nominal_value=1  temperatureCellModel_specify=on  temperatureCellModel_priority=High  temperatureCellModel=ModuleAssembly3.Module1.temperatureCellModel K  temperatureCellModel_nominal_specify=off  temperatureCellModel_nominal_unit=K  temperatureCellModel_nominal_value=1  vParallelAssembly_specify=on  vParallelAssembly_priority=None  vParallelAssembly=ModuleAssembly3.Module1.vParallelAssembly V  vParallelAssembly_nominal_specify=off  vParallelAssembly_nominal_unit=V  vParallelAssembly_nominal_value=1  socParallelAssembly_specify=on  socParallelAssembly_priority=None  socParallelAssembly=ModuleAssembly3.Module1.socParallelAssembly  socParallelAssembly_nominal_specify=off  socParallelAssembly_nominal_unit=1  socParallelAssembly_nominal_value=1
      settings: InternalSimscapePortConfiguration="{\"Bottom\":[{\"id\":\"n\",\"label\":\"-\",\"type\":\"foundation.electrical.electrical\"}],\"Left\":[{\"id\":\"ClntH\",\"label\":\"CH\",\"type\":\"foundation.thermal.thermal\"}],\"Right\":[],\"Top\":[{\"id\":\"p\",\"label\":\"+\",\"type\":\"foundation.electrical.electrical\"}]}"
  Module1_outputs : SimscapeProbe  BoundBlock=179  Variables={iCellModel, numCyclesCellModel, socCellModel, socParallelAssembly, temperatureCellModel, vCellModel, vParallelAssembly}
  Module2 : batt_packBTMSExampleLib_lib/Modules/ModuleType1  SOC_vec=ModuleType1.SOC_vec  T_vec=ModuleType1.T_vec K  V0_mat=ModuleType1.V0_mat V  V_range=ModuleType1.V_range V  R0_mat=ModuleType1.R0_mat Ohm  AH=ModuleType1.AH A*hr  extrapolation_option=simscape.enum.extrapolation.nearest  thermal_mass=ModuleType1.thermal_mass J/K  CoolantThermalPathResistance=ModuleType1.CoolantThermalPathResistance K/W  P=3  S=11  iCellModel_specify=on  iCellModel_priority=None  iCellModel=ModuleAssembly3.Module2.iCellModel A  iCellModel_nominal_specify=off  iCellModel_nominal_unit=A  iCellModel_nominal_value=1  vCellModel_specify=on  vCellModel_priority=None  vCellModel=ModuleAssembly3.Module2.vCellModel V  vCellModel_nominal_specify=off  vCellModel_nominal_unit=V  vCellModel_nominal_value=1  socCellModel_specify=on  socCellModel_priority=High  socCellModel=ModuleAssembly3.Module2.socCellModel  socCellModel_nominal_specify=off  socCellModel_nominal_unit=1  socCellModel_nominal_value=1  numCyclesCellModel_specify=on  numCyclesCellModel_priority=High  numCyclesCellModel=ModuleAssembly3.Module2.numCyclesCellModel  numCyclesCellModel_nominal_specify=off  numCyclesCellModel_nominal_unit=1  numCyclesCellModel_nominal_value=1  temperatureCellModel_specify=on  temperatureCellModel_priority=High  temperatureCellModel=ModuleAssembly3.Module2.temperatureCellModel K  temperatureCellModel_nominal_specify=off  temperatureCellModel_nominal_unit=K  temperatureCellModel_nominal_value=1  vParallelAssembly_specify=on  vParallelAssembly_priority=None  vParallelAssembly=ModuleAssembly3.Module2.vParallelAssembly V  vParallelAssembly_nominal_specify=off  vParallelAssembly_nominal_unit=V  vParallelAssembly_nominal_value=1  socParallelAssembly_specify=on  socParallelAssembly_priority=None  socParallelAssembly=ModuleAssembly3.Module2.socParallelAssembly  socParallelAssembly_nominal_specify=off  socParallelAssembly_nominal_unit=1  socParallelAssembly_nominal_value=1
      settings: InternalSimscapePortConfiguration="{\"Bottom\":[{\"id\":\"n\",\"label\":\"-\",\"type\":\"foundation.electrical.electrical\"}],\"Left\":[{\"id\":\"ClntH\",\"label\":\"CH\",\"type\":\"foundation.thermal.thermal\"}],\"Right\":[],\"Top\":[{\"id\":\"p\",\"label\":\"+\",\"type\":\"foundation.electrical.electrical\"}]}"
  Module2_outputs : SimscapeProbe  BoundBlock=181  Variables={iCellModel, numCyclesCellModel, socCellModel, socParallelAssembly, temperatureCellModel, vCellModel, vParallelAssembly}
  iCellModelMux : Mux  Inputs=2
  numCyclesCellModelMux : Mux  Inputs=2
  socCellModelMux : Mux  Inputs=2
  socParallelAssemblyMux : Mux  Inputs=2
  temperatureCellModelMux : Mux  Inputs=2
  vCellModelMux : Mux  Inputs=2
  vParallelAssemblyMux : Mux  Inputs=2
  + : PMIOPort  Side=Left
  - : PMIOPort  Port=2  Side=Right
  ClntH : PMIOPort  Port=3  Side=Right
  iCellModel : Outport
  numCyclesCellModel : Outport  Port=2
  socCellModel : Outport  Port=3
  socParallelAssembly : Outport  Port=4
  temperatureCellModel : Outport  Port=5
  vCellModel : Outport  Port=6
  vParallelAssembly : Outport  Port=7
  wires:
  [vParallelAssembly2] -> vParallelAssemblyMux/2
  Module2_outputs/1 -> [iCellModel2]
  [vCellModel2] -> vCellModelMux/2
  Module2_outputs/2 -> [numCyclesCellModel2]
  [temperatureCellModel2] -> temperatureCellModelMux/2
  Module2_outputs/3 -> [socCellModel2]
  [socParallelAssembly2] -> socParallelAssemblyMux/2
  Module2_outputs/4 -> [socParallelAssembly2]
  [socCellModel2] -> socCellModelMux/2
  Module2_outputs/5 -> [temperatureCellModel2]
  [numCyclesCellModel2] -> numCyclesCellModelMux/2
  Module2_outputs/6 -> [vCellModel2]
  [iCellModel2] -> iCellModelMux/2
  Module2_outputs/7 -> [vParallelAssembly2]
  [vParallelAssembly1] -> vParallelAssemblyMux/1
  vParallelAssemblyMux/1 -> vParallelAssembly/1
  Module1_outputs/1 -> [iCellModel1]
  [vCellModel1] -> vCellModelMux/1
  vCellModelMux/1 -> vCellModel/1
  Module1_outputs/2 -> [numCyclesCellModel1]
  [temperatureCellModel1] -> temperatureCellModelMux/1
  temperatureCellModelMux/1 -> temperatureCellModel/1
  Module1_outputs/3 -> [socCellModel1]
  [socParallelAssembly1] -> socParallelAssemblyMux/1
  socParallelAssemblyMux/1 -> socParallelAssembly/1
  Module1_outputs/4 -> [socParallelAssembly1]
  [socCellModel1] -> socCellModelMux/1
  socCellModelMux/1 -> socCellModel/1
  Module1_outputs/5 -> [temperatureCellModel1]
  [numCyclesCellModel1] -> numCyclesCellModelMux/1
  numCyclesCellModelMux/1 -> numCyclesCellModel/1
  Module1_outputs/6 -> [vCellModel1]
  [iCellModel1] -> iCellModelMux/1
  iCellModelMux/1 -> iCellModel/1
  Module1_outputs/7 -> [vParallelAssembly1]
  connections:
  ClntH_To_2/LConn1 -- Module2/LConn1
  ClntH_From_2/LConn1 -- ClntH_From_1/LConn1 -- ClntH/RConn1
  ClntH_To_1/LConn1 -- Module1/LConn1
  Module2/RConn1 -- -/RConn1
  Module1/LConn2 -- +/RConn1
  Module2/LConn2 -- Module1/RConn1
